simulink model "task_2e_simulink"  (R2014b)
settings: Solver=ode45  StartTime=0.0  StopTime=450  RelTol=1e-3
values from neighbouring files (symbols this model uses):
  Kp_chi = 1    [task_2e_different_kp_values.m]
undefined symbols (not defined in the file or in its folder): a_phi_1, a_phi_2, g, Kd_phi, Ki_chi, Kp_phi, Vg
settings Model: Creator=Ultrawack  LastModifiedBy=Ultrawack

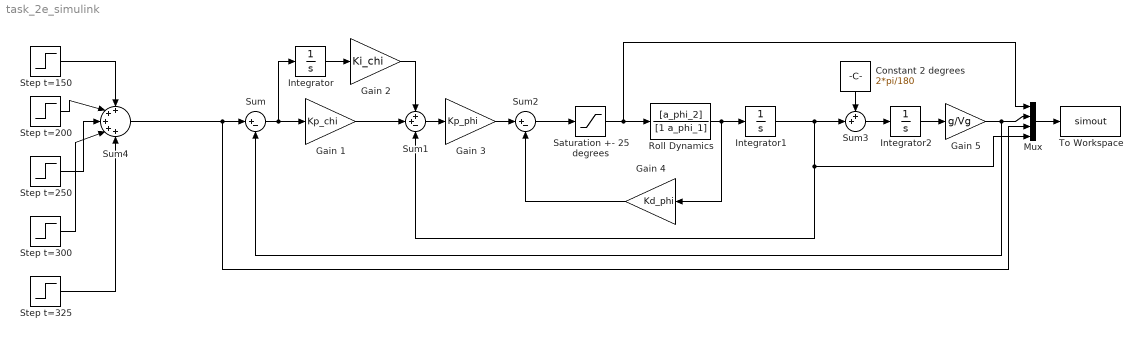
== system task_2e_simulink ==
  Constant 2 degrees : Constant  Value=2*pi/180
  Gain 1 : Gain  Gain=Kp_chi
  Gain 2 : Gain  Gain=Ki_chi
  Gain 3 : Gain  Gain=Kp_phi
  Gain 4 : Gain  Gain=Kd_phi
  Gain 5 : Gain  Gain=g/Vg
  Integrator : Integrator
  Integrator1 : Integrator
  Integrator2 : Integrator
  Mux : Mux
  Roll Dynamics : TransferFcn  Numerator=[a_phi_2]  Denominator=[1 a_phi_1]
  Saturation +- 25 degrees : Saturate  UpperLimit=25*pi/180  LowerLimit=-25*pi/180
  Step t=150 : Step  Time=100  After=0.20  SampleTime=0
  Step t=200 : Step  Time=200  After=0.15  SampleTime=0
  Step t=250 : Step  Time=220  After=0.20  SampleTime=0
  Step t=300 : Step  Time=300  After=0.25  SampleTime=0
  Step t=325 : Step  Time=375  After=-0.10  SampleTime=0
  Sum : Sum  Inputs=|+-
  Sum1 : Sum  Inputs=++-
  Sum2 : Sum  Inputs=|+-
  Sum3 : Sum  Inputs=++|
  Sum4 : Sum  Inputs=+++++
  To Workspace : ToWorkspace  VariableName=simout  SampleTime=-1
  wires:
  Sum/1 -> Integrator/1, Gain 1/1
  Sum1/1 -> Gain 3/1
  Gain 1/1 -> Sum1/2
  Integrator/1 -> Gain 2/1
  Gain 2/1 -> Sum1/1
  Gain 3/1 -> Sum2/1
  Gain 4/1 -> Sum2/2
  Roll Dynamics/1 -> Integrator1/1, Gain 4/1
  Integrator1/1 -> Sum3/2, Mux/4, Sum1/3
  Gain 5/1 -> Mux/2, Sum/2
  Constant 2 degrees/1 -> Sum3/1
  Saturation +- 25 degrees/1 -> Mux/1, Roll Dynamics/1
  Sum3/1 -> Integrator2/1
  Integrator2/1 -> Gain 5/1
  Sum2/1 -> Saturation +- 25 degrees/1
  Mux/1 -> To Workspace/1
  Step t=150/1 -> Sum4/1
  Step t=200/1 -> Sum4/2
  Step t=250/1 -> Sum4/3
  Step t=300/1 -> Sum4/4
  Step t=325/1 -> Sum4/5
  Sum4/1 -> Mux/3, Sum/1
